simulink library "halout"  (R2021b)
settings: Solver=VariableStepAuto  StartTime=0.0  StopTime=10.0  RelTol=1e-3
undefined symbols (not defined in the file): C_TASK_5MS_S, FALSE, KHAL_CAN1FDAPS3E2E_flg, KHAL_CAN1FDAPS3TxReq_flg, KHAL_CAN1FDVCU2E2E_flg, KHAL_CAN1FDVCU2TxReq_flg, KHAL_CAN1FDVCU3E2E_flg, KHAL_CAN1FDVCU3TxReq_flg, KHAL_CAN1TxReq_flg, KHAL_CAN2TxReq_flg, KHAL_CAN3FDVCU1TxReq_flg, KHAL_CAN3FDVCU2E2E_flg, KHAL_CAN3FDVCU2TxReq_flg, KHAL_CAN3TxReq_flg, KHAL_CAN4FDVCU1E2E_flg, KHAL_CAN4FDVCU1TxReq_flg, KHAL_CAN4TxReq_flg, KHAL_CAN5TxReq_flg, ONE_INT, TRUE, ZERO_INT
libraries: FVT_lib x383, simulink x179
(part 17 of 20)

== system halout/HAL_OUT/CAN3/FD_VCU2_0x154/Byte_15 ==
  Rr_TMTqReq : Inport
  BitwiseOR : simulink/Logic and Bit Operations/Bitwise Operator  logicop=OR  UseBitMask=off  BitMask=bin2dec('11011001')  BitMaskRealWorld=Stored Integer
  SignalPack : FVT_lib/hal/SignalPack  RightShiftCnt=0  BitMask=2^8-1  LeftShiftCnt=0
  UnitConverter : DataTypeConversion  OutDataTypeStr=uint8  RndMeth=Round
  UnitConverter1 : DataTypeConversion  OutDataTypeStr=uint16  RndMeth=Round
  convert_out : FVT_lib/hal/convert_out  gain=1  offset=-530
  Byte_15 : Outport
  wires:
  BitwiseOR/1 -> Byte_15/1
  UnitConverter/1 -> BitwiseOR/1
  SignalPack/1 -> UnitConverter/1
  UnitConverter1/1 -> SignalPack/1
  convert_out/1 -> UnitConverter1/1
  Rr_TMTqReq/1 -> convert_out/1

== system halout/HAL_OUT/CAN3/FD_VCU2_0x154/Byte_16 ==
  Fr_TMTqReq : Inport
  BitwiseOR : simulink/Logic and Bit Operations/Bitwise Operator  logicop=OR  UseBitMask=off  BitMask=bin2dec('11011001')  BitMaskRealWorld=Stored Integer
  SignalPack : FVT_lib/hal/SignalPack  RightShiftCnt=8  BitMask=2^8-1  LeftShiftCnt=0
  UnitConverter : DataTypeConversion  OutDataTypeStr=uint8  RndMeth=Round
  UnitConverter1 : DataTypeConversion  OutDataTypeStr=uint16  RndMeth=Round
  convert_out : FVT_lib/hal/convert_out  gain=1  offset=-530
  Byte_16 : Outport
  wires:
  BitwiseOR/1 -> Byte_16/1
  UnitConverter/1 -> BitwiseOR/1
  SignalPack/1 -> UnitConverter/1
  UnitConverter1/1 -> SignalPack/1
  convert_out/1 -> UnitConverter1/1
  Fr_TMTqReq/1 -> convert_out/1

== system halout/HAL_OUT/CAN3/FD_VCU2_0x154/Byte_17 ==
  Fr_TMTqReq : Inport
  BitwiseOR : simulink/Logic and Bit Operations/Bitwise Operator  logicop=OR  UseBitMask=off  BitMask=bin2dec('11011001')  BitMaskRealWorld=Stored Integer
  SignalPack : FVT_lib/hal/SignalPack  RightShiftCnt=0  BitMask=2^8-1  LeftShiftCnt=0
  UnitConverter : DataTypeConversion  OutDataTypeStr=uint8  RndMeth=Round
  UnitConverter1 : DataTypeConversion  OutDataTypeStr=uint16  RndMeth=Round
  convert_out : FVT_lib/hal/convert_out  gain=1  offset=-530
  Byte_17 : Outport
  wires:
  BitwiseOR/1 -> Byte_17/1
  UnitConverter/1 -> BitwiseOR/1
  SignalPack/1 -> UnitConverter/1
  UnitConverter1/1 -> SignalPack/1
  convert_out/1 -> UnitConverter1/1
  Fr_TMTqReq/1 -> convert_out/1

== system halout/HAL_OUT/CAN3/FD_VCU2_0x154/Byte_18 ==
  Fr_IdcMax : Inport
  BitwiseOR : simulink/Logic and Bit Operations/Bitwise Operator  logicop=OR  UseBitMask=off  BitMask=bin2dec('11011001')  BitMaskRealWorld=Stored Integer
  SignalPack : FVT_lib/hal/SignalPack  RightShiftCnt=4  BitMask=2^8-1  LeftShiftCnt=0
  UnitConverter : DataTypeConversion  OutDataTypeStr=uint8  RndMeth=Round
  UnitConverter1 : DataTypeConversion  OutDataTypeStr=uint16  RndMeth=Round
  Byte_18 : Outport
  wires:
  BitwiseOR/1 -> Byte_18/1
  UnitConverter/1 -> BitwiseOR/1
  SignalPack/1 -> UnitConverter/1
  UnitConverter1/1 -> SignalPack/1
  Fr_IdcMax/1 -> UnitConverter1/1

== system halout/HAL_OUT/CAN3/FD_VCU2_0x154/Byte_19 ==
  Fr_IdcMax : Inport
  Fr_IdcMin : Inport  Port=2
  BitwiseOR : simulink/Logic and Bit Operations/Bitwise Operator  logicop=OR  UseBitMask=off  NumInputPorts=2  BitMask=bin2dec('11011001')  BitMaskRealWorld=Stored Integer
  SignalPack : FVT_lib/hal/SignalPack  RightShiftCnt=0  BitMask=2^4-1  LeftShiftCnt=4
  SignalPack1 : FVT_lib/hal/SignalPack  RightShiftCnt=8  BitMask=2^4-1  LeftShiftCnt=0
  UnitConverter : DataTypeConversion  OutDataTypeStr=uint8  RndMeth=Round
  UnitConverter1 : DataTypeConversion  OutDataTypeStr=uint16  RndMeth=Round
  UnitConverter2 : DataTypeConversion  OutDataTypeStr=uint8  RndMeth=Round
  UnitConverter3 : DataTypeConversion  OutDataTypeStr=uint16  RndMeth=Round
  convert_out : FVT_lib/hal/convert_out  gain=1  offset=-1022
  Byte_19 : Outport
  wires:
  BitwiseOR/1 -> Byte_19/1
  UnitConverter/1 -> BitwiseOR/1
  SignalPack/1 -> UnitConverter/1
  UnitConverter1/1 -> SignalPack/1
  Fr_IdcMax/1 -> UnitConverter1/1
  UnitConverter2/1 -> BitwiseOR/2
  SignalPack1/1 -> UnitConverter2/1
  UnitConverter3/1 -> SignalPack1/1
  convert_out/1 -> UnitConverter3/1
  Fr_IdcMin/1 -> convert_out/1

== system halout/HAL_OUT/CAN3/FD_VCU2_0x154/Byte_2 ==
  Rr_IdcMax : Inport
  BitwiseOR : simulink/Logic and Bit Operations/Bitwise Operator  logicop=OR  UseBitMask=off  BitMask=bin2dec('11011001')  BitMaskRealWorld=Stored Integer
  SignalPack : FVT_lib/hal/SignalPack  RightShiftCnt=4  BitMask=2^8-1  LeftShiftCnt=0
  UnitConverter : DataTypeConversion  OutDataTypeStr=uint8  RndMeth=Round
  UnitConverter1 : DataTypeConversion  OutDataTypeStr=uint16  RndMeth=Round
  Byte_2 : Outport
  wires:
  BitwiseOR/1 -> Byte_2/1
  UnitConverter/1 -> BitwiseOR/1
  SignalPack/1 -> UnitConverter/1
  UnitConverter1/1 -> SignalPack/1
  Rr_IdcMax/1 -> UnitConverter1/1

== system halout/HAL_OUT/CAN3/FD_VCU2_0x154/Byte_20 ==
  Fr_IdcMin : Inport
  BitwiseOR : simulink/Logic and Bit Operations/Bitwise Operator  logicop=OR  UseBitMask=off  BitMask=bin2dec('11011001')  BitMaskRealWorld=Stored Integer
  SignalPack : FVT_lib/hal/SignalPack  RightShiftCnt=0  BitMask=2^8-1  LeftShiftCnt=0
  UnitConverter : DataTypeConversion  OutDataTypeStr=uint8  RndMeth=Round
  UnitConverter1 : DataTypeConversion  OutDataTypeStr=uint16  RndMeth=Round
  convert_out : FVT_lib/hal/convert_out  gain=1  offset=-1022
  Byte_20 : Outport
  wires:
  BitwiseOR/1 -> Byte_20/1
  UnitConverter/1 -> BitwiseOR/1
  SignalPack/1 -> UnitConverter/1
  UnitConverter1/1 -> SignalPack/1
  convert_out/1 -> UnitConverter1/1
  Fr_IdcMin/1 -> convert_out/1

== system halout/HAL_OUT/CAN3/FD_VCU2_0x154/Byte_21 ==
  Fr_TorqMax : Inport
  BitwiseOR : simulink/Logic and Bit Operations/Bitwise Operator  logicop=OR  UseBitMask=off  BitMask=bin2dec('11011001')  BitMaskRealWorld=Stored Integer
  SignalPack : FVT_lib/hal/SignalPack  RightShiftCnt=4  BitMask=2^8-1  LeftShiftCnt=0
  UnitConverter : DataTypeConversion  OutDataTypeStr=uint8  RndMeth=Round
  UnitConverter1 : DataTypeConversion  OutDataTypeStr=uint16  RndMeth=Round
  Byte_21 : Outport
  wires:
  BitwiseOR/1 -> Byte_21/1
  UnitConverter/1 -> BitwiseOR/1
  SignalPack/1 -> UnitConverter/1
  UnitConverter1/1 -> SignalPack/1
  Fr_TorqMax/1 -> UnitConverter1/1

== system halout/HAL_OUT/CAN3/FD_VCU2_0x154/Byte_22 ==
  Fr_TorqMax : Inport
  Fr_TorqMin : Inport  Port=2
  BitwiseOR : simulink/Logic and Bit Operations/Bitwise Operator  logicop=OR  UseBitMask=off  NumInputPorts=2  BitMask=bin2dec('11011001')  BitMaskRealWorld=Stored Integer
  SignalPack : FVT_lib/hal/SignalPack  RightShiftCnt=0  BitMask=2^4-1  LeftShiftCnt=4
  SignalPack1 : FVT_lib/hal/SignalPack  RightShiftCnt=8  BitMask=2^4-1  LeftShiftCnt=0
  UnitConverter : DataTypeConversion  OutDataTypeStr=uint8  RndMeth=Round
  UnitConverter1 : DataTypeConversion  OutDataTypeStr=uint16  RndMeth=Round
  UnitConverter2 : DataTypeConversion  OutDataTypeStr=uint8  RndMeth=Round
  UnitConverter3 : DataTypeConversion  OutDataTypeStr=uint16  RndMeth=Round
  convert_out : FVT_lib/hal/convert_out  gain=1  offset=-1022
  Byte_22 : Outport
  wires:
  BitwiseOR/1 -> Byte_22/1
  UnitConverter/1 -> BitwiseOR/1
  SignalPack/1 -> UnitConverter/1
  UnitConverter1/1 -> SignalPack/1
  Fr_TorqMax/1 -> UnitConverter1/1
  UnitConverter2/1 -> BitwiseOR/2
  SignalPack1/1 -> UnitConverter2/1
  UnitConverter3/1 -> SignalPack1/1
  convert_out/1 -> UnitConverter3/1
  Fr_TorqMin/1 -> convert_out/1

== system halout/HAL_OUT/CAN3/FD_VCU2_0x154/Byte_23 ==
  Fr_TorqMin : Inport
  BitwiseOR : simulink/Logic and Bit Operations/Bitwise Operator  logicop=OR  UseBitMask=off  BitMask=bin2dec('11011001')  BitMaskRealWorld=Stored Integer
  SignalPack : FVT_lib/hal/SignalPack  RightShiftCnt=0  BitMask=2^8-1  LeftShiftCnt=0
  UnitConverter : DataTypeConversion  OutDataTypeStr=uint8  RndMeth=Round
  UnitConverter1 : DataTypeConversion  OutDataTypeStr=uint16  RndMeth=Round
  convert_out : FVT_lib/hal/convert_out  gain=1  offset=-1022
  Byte_23 : Outport
  wires:
  BitwiseOR/1 -> Byte_23/1
  UnitConverter/1 -> BitwiseOR/1
  SignalPack/1 -> UnitConverter/1
  UnitConverter1/1 -> SignalPack/1
  convert_out/1 -> UnitConverter1/1
  Fr_TorqMin/1 -> convert_out/1

== system halout/HAL_OUT/CAN3/FD_VCU2_0x154/Byte_3 ==
  Rr_IdcMax : Inport
  Rr_IdcMin : Inport  Port=2
  BitwiseOR : simulink/Logic and Bit Operations/Bitwise Operator  logicop=OR  UseBitMask=off  NumInputPorts=2  BitMask=bin2dec('11011001')  BitMaskRealWorld=Stored Integer
  SignalPack : FVT_lib/hal/SignalPack  RightShiftCnt=0  BitMask=2^4-1  LeftShiftCnt=4
  SignalPack1 : FVT_lib/hal/SignalPack  RightShiftCnt=8  BitMask=2^4-1  LeftShiftCnt=0
  UnitConverter : DataTypeConversion  OutDataTypeStr=uint8  RndMeth=Round
  UnitConverter1 : DataTypeConversion  OutDataTypeStr=uint16  RndMeth=Round
  UnitConverter2 : DataTypeConversion  OutDataTypeStr=uint8  RndMeth=Round
  UnitConverter3 : DataTypeConversion  OutDataTypeStr=uint16  RndMeth=Round
  convert_out : FVT_lib/hal/convert_out  gain=1  offset=-1022
  Byte_3 : Outport
  wires:
  BitwiseOR/1 -> Byte_3/1
  UnitConverter/1 -> BitwiseOR/1
  SignalPack/1 -> UnitConverter/1
  UnitConverter1/1 -> SignalPack/1
  Rr_IdcMax/1 -> UnitConverter1/1
  UnitConverter2/1 -> BitwiseOR/2
  SignalPack1/1 -> UnitConverter2/1
  UnitConverter3/1 -> SignalPack1/1
  convert_out/1 -> UnitConverter3/1
  Rr_IdcMin/1 -> convert_out/1

== system halout/HAL_OUT/CAN3/FD_VCU2_0x154/Byte_4 ==
  Rr_IdcMin : Inport
  BitwiseOR : simulink/Logic and Bit Operations/Bitwise Operator  logicop=OR  UseBitMask=off  BitMask=bin2dec('11011001')  BitMaskRealWorld=Stored Integer
  SignalPack : FVT_lib/hal/SignalPack  RightShiftCnt=0  BitMask=2^8-1  LeftShiftCnt=0
  UnitConverter : DataTypeConversion  OutDataTypeStr=uint8  RndMeth=Round
  UnitConverter1 : DataTypeConversion  OutDataTypeStr=uint16  RndMeth=Round
  convert_out : FVT_lib/hal/convert_out  gain=1  offset=-1022
  Byte_4 : Outport
  wires:
  BitwiseOR/1 -> Byte_4/1
  UnitConverter/1 -> BitwiseOR/1
  SignalPack/1 -> UnitConverter/1
  UnitConverter1/1 -> SignalPack/1
  convert_out/1 -> UnitConverter1/1
  Rr_IdcMin/1 -> convert_out/1

== system halout/HAL_OUT/CAN3/FD_VCU2_0x154/Byte_5 ==
  Rr_TorqMax : Inport
  BitwiseOR : simulink/Logic and Bit Operations/Bitwise Operator  logicop=OR  UseBitMask=off  BitMask=bin2dec('11011001')  BitMaskRealWorld=Stored Integer
  SignalPack : FVT_lib/hal/SignalPack  RightShiftCnt=4  BitMask=2^8-1  LeftShiftCnt=0
  UnitConverter : DataTypeConversion  OutDataTypeStr=uint8  RndMeth=Round
  UnitConverter1 : DataTypeConversion  OutDataTypeStr=uint16  RndMeth=Round
  Byte_5 : Outport
  wires:
  BitwiseOR/1 -> Byte_5/1
  UnitConverter/1 -> BitwiseOR/1
  SignalPack/1 -> UnitConverter/1
  UnitConverter1/1 -> SignalPack/1
  Rr_TorqMax/1 -> UnitConverter1/1

== system halout/HAL_OUT/CAN3/FD_VCU2_0x154/Byte_6 ==
  Rr_TorqMax : Inport
  Rr_TorqMin : Inport  Port=2
  BitwiseOR : simulink/Logic and Bit Operations/Bitwise Operator  logicop=OR  UseBitMask=off  NumInputPorts=2  BitMask=bin2dec('11011001')  BitMaskRealWorld=Stored Integer
  SignalPack : FVT_lib/hal/SignalPack  RightShiftCnt=0  BitMask=2^4-1  LeftShiftCnt=4
  SignalPack1 : FVT_lib/hal/SignalPack  RightShiftCnt=8  BitMask=2^4-1  LeftShiftCnt=0
  UnitConverter : DataTypeConversion  OutDataTypeStr=uint8  RndMeth=Round
  UnitConverter1 : DataTypeConversion  OutDataTypeStr=uint16  RndMeth=Round
  UnitConverter2 : DataTypeConversion  OutDataTypeStr=uint8  RndMeth=Round
  UnitConverter3 : DataTypeConversion  OutDataTypeStr=uint16  RndMeth=Round
  convert_out : FVT_lib/hal/convert_out  gain=1  offset=-1022
  Byte_6 : Outport
  wires:
  BitwiseOR/1 -> Byte_6/1
  UnitConverter/1 -> BitwiseOR/1
  SignalPack/1 -> UnitConverter/1
  UnitConverter1/1 -> SignalPack/1
  Rr_TorqMax/1 -> UnitConverter1/1
  UnitConverter2/1 -> BitwiseOR/2
  SignalPack1/1 -> UnitConverter2/1
  UnitConverter3/1 -> SignalPack1/1
  convert_out/1 -> UnitConverter3/1
  Rr_TorqMin/1 -> convert_out/1

== system halout/HAL_OUT/CAN3/FD_VCU2_0x154/Byte_7 ==
  Rr_TorqMin : Inport
  BitwiseOR : simulink/Logic and Bit Operations/Bitwise Operator  logicop=OR  UseBitMask=off  BitMask=bin2dec('11011001')  BitMaskRealWorld=Stored Integer
  SignalPack : FVT_lib/hal/SignalPack  RightShiftCnt=0  BitMask=2^8-1  LeftShiftCnt=0
  UnitConverter : DataTypeConversion  OutDataTypeStr=uint8  RndMeth=Round
  UnitConverter1 : DataTypeConversion  OutDataTypeStr=uint16  RndMeth=Round
  convert_out : FVT_lib/hal/convert_out  gain=1  offset=-1022
  Byte_7 : Outport
  wires:
  BitwiseOR/1 -> Byte_7/1
  UnitConverter/1 -> BitwiseOR/1
  SignalPack/1 -> UnitConverter/1
  UnitConverter1/1 -> SignalPack/1
  convert_out/1 -> UnitConverter1/1
  Rr_TorqMin/1 -> convert_out/1

== system halout/HAL_OUT/CAN3/FD_VCU2_0x154/Byte_8 ==
  Rr_UdcMax : Inport
  BitwiseOR : simulink/Logic and Bit Operations/Bitwise Operator  logicop=OR  UseBitMask=off  BitMask=bin2dec('11011001')  BitMaskRealWorld=Stored Integer
  SignalPack : FVT_lib/hal/SignalPack  RightShiftCnt=4  BitMask=2^8-1  LeftShiftCnt=0
  UnitConverter : DataTypeConversion  OutDataTypeStr=uint8  RndMeth=Round
  UnitConverter1 : DataTypeConversion  OutDataTypeStr=uint16  RndMeth=Round
  Byte_8 : Outport
  wires:
  BitwiseOR/1 -> Byte_8/1
  UnitConverter/1 -> BitwiseOR/1
  SignalPack/1 -> UnitConverter/1
  UnitConverter1/1 -> SignalPack/1
  Rr_UdcMax/1 -> UnitConverter1/1

== system halout/HAL_OUT/CAN3/FD_VCU2_0x154/Byte_9 ==
  Rr_UdcMax : Inport
  Rr_UdcMin : Inport  Port=2
  BitwiseOR : simulink/Logic and Bit Operations/Bitwise Operator  logicop=OR  UseBitMask=off  NumInputPorts=2  BitMask=bin2dec('11011001')  BitMaskRealWorld=Stored Integer
  SignalPack : FVT_lib/hal/SignalPack  RightShiftCnt=0  BitMask=2^4-1  LeftShiftCnt=4
  SignalPack1 : FVT_lib/hal/SignalPack  RightShiftCnt=8  BitMask=2^4-1  LeftShiftCnt=0
  UnitConverter : DataTypeConversion  OutDataTypeStr=uint8  RndMeth=Round
  UnitConverter1 : DataTypeConversion  OutDataTypeStr=uint16  RndMeth=Round
  UnitConverter2 : DataTypeConversion  OutDataTypeStr=uint8  RndMeth=Round
  UnitConverter3 : DataTypeConversion  OutDataTypeStr=uint16  RndMeth=Round
  Byte_9 : Outport
  wires:
  BitwiseOR/1 -> Byte_9/1
  UnitConverter/1 -> BitwiseOR/1
  SignalPack/1 -> UnitConverter/1
  UnitConverter1/1 -> SignalPack/1
  Rr_UdcMax/1 -> UnitConverter1/1
  UnitConverter2/1 -> BitwiseOR/2
  SignalPack1/1 -> UnitConverter2/1
  UnitConverter3/1 -> SignalPack1/1
  Rr_UdcMin/1 -> UnitConverter3/1

== system halout/HAL_OUT/CAN3/FD_VCU2_0x154/CSVCU2CAN1 ==
  CSVCU2CAN1 : Inport
  Data Type Conversion : DataTypeConversion  OutDataTypeStr=uint8  RndMeth=Round
  CAN3_CS_VCU2_CAN1 : Outport
  wires:
  Data Type Conversion/1 -> CAN3_CS_VCU2_CAN1/1
  CSVCU2CAN1/1 -> Data Type Conversion/1

== system halout/HAL_OUT/CAN3/FD_VCU2_0x154/FrIdcMax ==
  FrIdcMax : Inport
  Data Type Conversion : DataTypeConversion  OutDataTypeStr=uint16  RndMeth=Round
  CAN3_Fr_IdcMax : Outport
  wires:
  Data Type Conversion/1 -> CAN3_Fr_IdcMax/1
  FrIdcMax/1 -> Data Type Conversion/1

== system halout/HAL_OUT/CAN3/FD_VCU2_0x154/FrIdcMin ==
  FrIdcMin : Inport
  Data Type Conversion : DataTypeConversion  OutDataTypeStr=uint16  RndMeth=Round
  convert_out : FVT_lib/hal/convert_out  gain=1  offset=-1022
  CAN3_Fr_IdcMin : Outport
  wires:
  Data Type Conversion/1 -> CAN3_Fr_IdcMin/1
  convert_out/1 -> Data Type Conversion/1
  FrIdcMin/1 -> convert_out/1

== system halout/HAL_OUT/CAN3/FD_VCU2_0x154/FrTMTqReq ==
  FrTMTqReq : Inport
  Data Type Conversion : DataTypeConversion  OutDataTypeStr=uint16  RndMeth=Round
  convert_out : FVT_lib/hal/convert_out  gain=1  offset=-530
  CAN3_Fr_TMTqReq : Outport
  wires:
  Data Type Conversion/1 -> CAN3_Fr_TMTqReq/1
  convert_out/1 -> Data Type Conversion/1
  FrTMTqReq/1 -> convert_out/1

== system halout/HAL_OUT/CAN3/FD_VCU2_0x154/FrTorqMax ==
  FrTorqMax : Inport
  Data Type Conversion : DataTypeConversion  OutDataTypeStr=uint16  RndMeth=Round
  CAN3_Fr_TorqMax : Outport
  wires:
  Data Type Conversion/1 -> CAN3_Fr_TorqMax/1
  FrTorqMax/1 -> Data Type Conversion/1

== system halout/HAL_OUT/CAN3/FD_VCU2_0x154/FrTorqMin ==
  FrTorqMin : Inport
  Data Type Conversion : DataTypeConversion  OutDataTypeStr=uint16  RndMeth=Round
  convert_out : FVT_lib/hal/convert_out  gain=1  offset=-1022
  CAN3_Fr_TorqMin : Outport
  wires:
  Data Type Conversion/1 -> CAN3_Fr_TorqMin/1
  convert_out/1 -> Data Type Conversion/1
  FrTorqMin/1 -> convert_out/1

== system halout/HAL_OUT/CAN3/FD_VCU2_0x154/FrUdcMax ==
  FrUdcMax : Inport
  Data Type Conversion : DataTypeConversion  OutDataTypeStr=uint16  RndMeth=Round
  CAN3_Fr_UdcMax : Outport
  wires:
  Data Type Conversion/1 -> CAN3_Fr_UdcMax/1
  FrUdcMax/1 -> Data Type Conversion/1

== system halout/HAL_OUT/CAN3/FD_VCU2_0x154/FrUdcMin ==
  FrUdcMin : Inport
  Data Type Conversion : DataTypeConversion  OutDataTypeStr=uint16  RndMeth=Round
  CAN3_Fr_UdcMin : Outport
  wires:
  Data Type Conversion/1 -> CAN3_Fr_UdcMin/1
  FrUdcMin/1 -> Data Type Conversion/1

== system halout/HAL_OUT/CAN3/FD_VCU2_0x154/RCVCU2CAN1 ==
  RCVCU2CAN1 : Inport
  Data Type Conversion : DataTypeConversion  OutDataTypeStr=uint8  RndMeth=Round
  CAN3_RC_VCU2_CAN1 : Outport
  wires:
  Data Type Conversion/1 -> CAN3_RC_VCU2_CAN1/1
  RCVCU2CAN1/1 -> Data Type Conversion/1

== system halout/HAL_OUT/CAN3/FD_VCU2_0x154/RrIdcMax ==
  RrIdcMax : Inport
  Data Type Conversion : DataTypeConversion  OutDataTypeStr=uint16  RndMeth=Round
  CAN3_Rr_IdcMax : Outport
  wires:
  Data Type Conversion/1 -> CAN3_Rr_IdcMax/1
  RrIdcMax/1 -> Data Type Conversion/1

== system halout/HAL_OUT/CAN3/FD_VCU2_0x154/RrIdcMin ==
  RrIdcMin : Inport
  Data Type Conversion : DataTypeConversion  OutDataTypeStr=uint16  RndMeth=Round
  convert_out : FVT_lib/hal/convert_out  gain=1  offset=-1022
  CAN3_Rr_IdcMin : Outport
  wires:
  Data Type Conversion/1 -> CAN3_Rr_IdcMin/1
  convert_out/1 -> Data Type Conversion/1
  RrIdcMin/1 -> convert_out/1

== system halout/HAL_OUT/CAN3/FD_VCU2_0x154/RrTMTqReq ==
  RrTMTqReq : Inport
  Data Type Conversion : DataTypeConversion  OutDataTypeStr=uint16  RndMeth=Round
  convert_out : FVT_lib/hal/convert_out  gain=1  offset=-530
  CAN3_Rr_TMTqReq : Outport
  wires:
  Data Type Conversion/1 -> CAN3_Rr_TMTqReq/1
  convert_out/1 -> Data Type Conversion/1
  RrTMTqReq/1 -> convert_out/1

== system halout/HAL_OUT/CAN3/FD_VCU2_0x154/RrTorqMax ==
  RrTorqMax : Inport
  Data Type Conversion : DataTypeConversion  OutDataTypeStr=uint16  RndMeth=Round
  CAN3_Rr_TorqMax : Outport
  wires:
  Data Type Conversion/1 -> CAN3_Rr_TorqMax/1
  RrTorqMax/1 -> Data Type Conversion/1

== system halout/HAL_OUT/CAN3/FD_VCU2_0x154/RrTorqMin ==
  RrTorqMin : Inport
  Data Type Conversion : DataTypeConversion  OutDataTypeStr=uint16  RndMeth=Round
  convert_out : FVT_lib/hal/convert_out  gain=1  offset=-1022
  CAN3_Rr_TorqMin : Outport
  wires:
  Data Type Conversion/1 -> CAN3_Rr_TorqMin/1
  convert_out/1 -> Data Type Conversion/1
  RrTorqMin/1 -> convert_out/1

== system halout/HAL_OUT/CAN3/FD_VCU2_0x154/RrUdcMax ==
  RrUdcMax : Inport
  Data Type Conversion : DataTypeConversion  OutDataTypeStr=uint16  RndMeth=Round
  CAN3_Rr_UdcMax : Outport
  wires:
  Data Type Conversion/1 -> CAN3_Rr_UdcMax/1
  RrUdcMax/1 -> Data Type Conversion/1

== system halout/HAL_OUT/CAN3/FD_VCU2_0x154/RrUdcMin ==
  RrUdcMin : Inport
  Data Type Conversion : DataTypeConversion  OutDataTypeStr=uint16  RndMeth=Round
  CAN3_Rr_UdcMin : Outport
  wires:
  Data Type Conversion/1 -> CAN3_Rr_UdcMin/1
  RrUdcMin/1 -> Data Type Conversion/1

== system halout/HAL_OUT/CAN4/FD_DKC1_0x253/ApproachUnlockSW ==
  ApproachUnlockSW : Inport
  Data Type Conversion : DataTypeConversion  OutDataTypeStr=uint8  RndMeth=Round
  CAN4_Approach_Unlock_SW : Outport
  wires:
  Data Type Conversion/1 -> CAN4_Approach_Unlock_SW/1
  ApproachUnlockSW/1 -> Data Type Conversion/1

== system halout/HAL_OUT/CAN4/FD_DKC1_0x253/BrkPedalPos ==
  BrkPedalPos : Inport
  Data Type Conversion : DataTypeConversion  OutDataTypeStr=uint8  RndMeth=Round
  convert_out : FVT_lib/hal/convert_out  gain=0.4  offset=0
  CAN4_BrkPedalPos : Outport
  wires:
  Data Type Conversion/1 -> CAN4_BrkPedalPos/1
  convert_out/1 -> Data Type Conversion/1
  BrkPedalPos/1 -> convert_out/1

== system halout/HAL_OUT/CAN4/FD_DKC1_0x253/BrkPedalPosSta ==
  BrkPedalPosSta : Inport
  Data Type Conversion : DataTypeConversion  OutDataTypeStr=uint8  RndMeth=Round
  CAN4_BrkPedalPos_Sta : Outport
  wires:
  Data Type Conversion/1 -> CAN4_BrkPedalPos_Sta/1
  BrkPedalPosSta/1 -> Data Type Conversion/1

== system halout/HAL_OUT/CAN4/FD_DKC1_0x253/BrkSwSta ==
  BrkSwSta : Inport
  Data Type Conversion : DataTypeConversion  OutDataTypeStr=uint8  RndMeth=Round
  CAN4_BrkSw_Sta : Outport
  wires:
  Data Type Conversion/1 -> CAN4_BrkSw_Sta/1
  BrkSwSta/1 -> Data Type Conversion/1

== system halout/HAL_OUT/CAN4/FD_DKC1_0x253/BrkSwV ==
  BrkSwV : Inport
  Data Type Conversion : DataTypeConversion  OutDataTypeStr=uint8  RndMeth=Round
  CAN4_BrkSw_V : Outport
  wires:
  Data Type Conversion/1 -> CAN4_BrkSw_V/1
  BrkSwV/1 -> Data Type Conversion/1

== system halout/HAL_OUT/CAN4/FD_DKC1_0x253/DSEATantiset ==
  DSEATantiset : Inport
  Data Type Conversion : DataTypeConversion  OutDataTypeStr=uint8  RndMeth=Round
  CAN4_DSEAT_anti_set : Outport
  wires:
  Data Type Conversion/1 -> CAN4_DSEAT_anti_set/1
  DSEATantiset/1 -> Data Type Conversion/1

== system halout/HAL_OUT/CAN4/FD_DKC1_0x253/DSEATentryfunset ==
  DSEATentryfunset : Inport
  Data Type Conversion : DataTypeConversion  OutDataTypeStr=uint8  RndMeth=Round
  CAN4_DSEAT_entryfun_set : Outport
  wires:
  Data Type Conversion/1 -> CAN4_DSEAT_entryfun_set/1
  DSEATentryfunset/1 -> Data Type Conversion/1

== system halout/HAL_OUT/CAN4/FD_DKC1_0x253/DSEATventreq ==
  DSEATventreq : Inport
  Data Type Conversion : DataTypeConversion  OutDataTypeStr=uint8  RndMeth=Round
  CAN4_DSEAT_vent_req : Outport
  wires:
  Data Type Conversion/1 -> CAN4_DSEAT_vent_req/1
  DSEATventreq/1 -> Data Type Conversion/1

== system halout/HAL_OUT/CAN4/FD_DKC1_0x253/FDCBCMATCtrlCmd ==
  FDCBCMATCtrlCmd : Inport
  Data Type Conversion : DataTypeConversion  OutDataTypeStr=uint8  RndMeth=Round
  CAN4_FDC_BCM_ATCtrl_Cmd : Outport
  wires:
  Data Type Conversion/1 -> CAN4_FDC_BCM_ATCtrl_Cmd/1
  FDCBCMATCtrlCmd/1 -> Data Type Conversion/1

== system halout/HAL_OUT/CAN4/FD_DKC1_0x253/FDCBCMLockAlarmCmd ==
  FDCBCMLockAlarmCmd : Inport
  Data Type Conversion : DataTypeConversion  OutDataTypeStr=uint8  RndMeth=Round
  CAN4_FDC_BCM_LockAlarm_Cmd : Outport
  wires:
  Data Type Conversion/1 -> CAN4_FDC_BCM_LockAlarm_Cmd/1
  FDCBCMLockAlarmCmd/1 -> Data Type Conversion/1

== system halout/HAL_OUT/CAN4/FD_DKC1_0x253/FDCBCMOutModeCmd ==
  FDCBCMOutModeCmd : Inport
  Data Type Conversion : DataTypeConversion  OutDataTypeStr=uint8  RndMeth=Round
  CAN4_FDC_BCM_OutMode_Cmd : Outport
  wires:
  Data Type Conversion/1 -> CAN4_FDC_BCM_OutMode_Cmd/1
  FDCBCMOutModeCmd/1 -> Data Type Conversion/1

== system halout/HAL_OUT/CAN4/FD_DKC1_0x253/FDCTHCMACTInitialCmd ==
  FDCTHCMACTInitialCmd : Inport
  Data Type Conversion : DataTypeConversion  OutDataTypeStr=uint8  RndMeth=Round
  CAN4_FDC_THCM_ACTInitial_Cmd : Outport
  wires:
  Data Type Conversion/1 -> CAN4_FDC_THCM_ACTInitial_Cmd/1
  FDCTHCMACTInitialCmd/1 -> Data Type Conversion/1

== system halout/HAL_OUT/CAN4/FD_DKC1_0x253/HeadLampSW ==
  HeadLampSW : Inport
  Data Type Conversion : DataTypeConversion  OutDataTypeStr=uint8  RndMeth=Round
  CAN4_HeadLampSW : Outport
  wires:
  Data Type Conversion/1 -> CAN4_HeadLampSW/1
  HeadLampSW/1 -> Data Type Conversion/1

== system halout/HAL_OUT/CAN4/FD_DKC1_0x253/HoodLatchSW ==
  HoodLatchSW : Inport
  Data Type Conversion : DataTypeConversion  OutDataTypeStr=uint8  RndMeth=Round
  CAN4_Hood_Latch_SW : Outport
  wires:
  Data Type Conversion/1 -> CAN4_Hood_Latch_SW/1
  HoodLatchSW/1 -> Data Type Conversion/1

== system halout/HAL_OUT/CAN4/FD_DKC1_0x253/IVIISAOffsetSpd ==
  IVIISAOffsetSpd : Inport
  Data Type Conversion : DataTypeConversion  OutDataTypeStr=uint8  RndMeth=Round
  CAN4_IVI_ISA_OffsetSpd : Outport
  wires:
  Data Type Conversion/1 -> CAN4_IVI_ISA_OffsetSpd/1
  IVIISAOffsetSpd/1 -> Data Type Conversion/1

== system halout/HAL_OUT/CAN4/FD_DKC1_0x253/IVILocatedSTA ==
  IVILocatedSTA : Inport
  Data Type Conversion : DataTypeConversion  OutDataTypeStr=uint8  RndMeth=Round
  CAN4_IVI_Located_STA : Outport
  wires:
  Data Type Conversion/1 -> CAN4_IVI_Located_STA/1
  IVILocatedSTA/1 -> Data Type Conversion/1

== system halout/HAL_OUT/CAN4/FD_DKC1_0x253/IVIPTGModeSW ==
  IVIPTGModeSW : Inport
  Data Type Conversion : DataTypeConversion  OutDataTypeStr=uint8  RndMeth=Round
  CAN4_IVI_PTG_Mode_SW : Outport
  wires:
  Data Type Conversion/1 -> CAN4_IVI_PTG_Mode_SW/1
  IVIPTGModeSW/1 -> Data Type Conversion/1

== system halout/HAL_OUT/CAN4/FD_DKC1_0x253/IVIPTGOpenHeight ==
  IVIPTGOpenHeight : Inport
  Data Type Conversion : DataTypeConversion  OutDataTypeStr=uint8  RndMeth=Round
  CAN4_IVI_PTG_Open_Height : Outport
  wires:
  Data Type Conversion/1 -> CAN4_IVI_PTG_Open_Height/1
  IVIPTGOpenHeight/1 -> Data Type Conversion/1

== system halout/HAL_OUT/CAN4/FD_DKC1_0x253/IVIPTGStaSW ==
  IVIPTGStaSW : Inport
  Data Type Conversion : DataTypeConversion  OutDataTypeStr=uint8  RndMeth=Round
  CAN4_IVI_PTG_Sta_SW : Outport
  wires:
  Data Type Conversion/1 -> CAN4_IVI_PTG_Sta_SW/1
  IVIPTGStaSW/1 -> Data Type Conversion/1

== system halout/HAL_OUT/CAN4/FD_DKC1_0x253/IVIPTGUSStaSW ==
  IVIPTGUSStaSW : Inport
  Data Type Conversion : DataTypeConversion  OutDataTypeStr=uint8  RndMeth=Round
  CAN4_IVI_PTG_USSta_SW : Outport
  wires:
  Data Type Conversion/1 -> CAN4_IVI_PTG_USSta_SW/1
  IVIPTGUSStaSW/1 -> Data Type Conversion/1

== system halout/HAL_OUT/CAN4/FD_DKC1_0x253/IVITimeCheck ==
  IVITimeCheck : Inport
  Data Type Conversion : DataTypeConversion  OutDataTypeStr=uint8  RndMeth=Round
  CAN4_IVI_Time_Check : Outport
  wires:
  Data Type Conversion/1 -> CAN4_IVI_Time_Check/1
  IVITimeCheck/1 -> Data Type Conversion/1

== system halout/HAL_OUT/CAN4/FD_DKC1_0x253/IVITimeDay ==
  IVITimeDay : Inport
  Data Type Conversion : DataTypeConversion  OutDataTypeStr=uint8  RndMeth=Round
  CAN4_IVI_Time_Day : Outport
  wires:
  Data Type Conversion/1 -> CAN4_IVI_Time_Day/1
  IVITimeDay/1 -> Data Type Conversion/1

== system halout/HAL_OUT/CAN4/FD_DKC1_0x253/IVITimeHour ==
  IVITimeHour : Inport
  Data Type Conversion : DataTypeConversion  OutDataTypeStr=uint8  RndMeth=Round
  CAN4_IVI_Time_Hour : Outport
  wires:
  Data Type Conversion/1 -> CAN4_IVI_Time_Hour/1
  IVITimeHour/1 -> Data Type Conversion/1

== system halout/HAL_OUT/CAN4/FD_DKC1_0x253/IVITimeMinute ==
  IVITimeMinute : Inport
  Data Type Conversion : DataTypeConversion  OutDataTypeStr=uint8  RndMeth=Round
  CAN4_IVI_Time_Minute : Outport
  wires:
  Data Type Conversion/1 -> CAN4_IVI_Time_Minute/1
  IVITimeMinute/1 -> Data Type Conversion/1

== system halout/HAL_OUT/CAN4/FD_DKC1_0x253/IVITimeMonth ==
  IVITimeMonth : Inport
  Data Type Conversion : DataTypeConversion  OutDataTypeStr=uint8  RndMeth=Round
  CAN4_IVI_Time_Month : Outport
  wires:
  Data Type Conversion/1 -> CAN4_IVI_Time_Month/1
  IVITimeMonth/1 -> Data Type Conversion/1

== system halout/HAL_OUT/CAN4/FD_DKC1_0x253/IVITimeSecond ==
  IVITimeSecond : Inport
  Data Type Conversion : DataTypeConversion  OutDataTypeStr=uint8  RndMeth=Round
  CAN4_IVI_Time_Second : Outport
  wires:
  Data Type Conversion/1 -> CAN4_IVI_Time_Second/1
  IVITimeSecond/1 -> Data Type Conversion/1

== system halout/HAL_OUT/CAN4/FD_DKC1_0x253/IVITimeYear ==
  IVITimeYear : Inport
  Data Type Conversion : DataTypeConversion  OutDataTypeStr=uint8  RndMeth=Round
  convert_out : FVT_lib/hal/convert_out  gain=1  offset=2000
  CAN4_IVI_Time_Year : Outport
  wires:
  Data Type Conversion/1 -> CAN4_IVI_Time_Year/1
  convert_out/1 -> Data Type Conversion/1
  IVITimeYear/1 -> convert_out/1

== system halout/HAL_OUT/CAN4/FD_DKC1_0x253/LDrvCtrlCmd ==
  LDrvCtrlCmd : Inport
  Data Type Conversion : DataTypeConversion  OutDataTypeStr=uint8  RndMeth=Round
  CAN4_L_Drv_CtrlCmd : Outport
  wires:
  Data Type Conversion/1 -> CAN4_L_Drv_CtrlCmd/1
  LDrvCtrlCmd/1 -> Data Type Conversion/1

== system halout/HAL_OUT/CAN4/FD_DKC1_0x253/LPasCtrlCmd ==
  LPasCtrlCmd : Inport
  Data Type Conversion : DataTypeConversion  OutDataTypeStr=uint8  RndMeth=Round
  CAN4_L_Pas_CtrlCmd : Outport
  wires:
  Data Type Conversion/1 -> CAN4_L_Pas_CtrlCmd/1
  LPasCtrlCmd/1 -> Data Type Conversion/1

== system halout/HAL_OUT/CAN4/FD_DKC1_0x253/LRLDCtrlCmd ==
  LRLDCtrlCmd : Inport
  Data Type Conversion : DataTypeConversion  OutDataTypeStr=uint8  RndMeth=Round
  CAN4_L_RLD_CtrlCmd : Outport
  wires:
  Data Type Conversion/1 -> CAN4_L_RLD_CtrlCmd/1
  LRLDCtrlCmd/1 -> Data Type Conversion/1

== system halout/HAL_OUT/CAN4/FD_DKC1_0x253/LRRDCtrlCmd ==
  LRRDCtrlCmd : Inport
  Data Type Conversion : DataTypeConversion  OutDataTypeStr=uint8  RndMeth=Round
  CAN4_L_RRD_CtrlCmd : Outport
  wires:
  Data Type Conversion/1 -> CAN4_L_RRD_CtrlCmd/1
  LRRDCtrlCmd/1 -> Data Type Conversion/1

== system halout/HAL_OUT/CAN4/FD_DKC1_0x253/MCPressure ==
  MCPressure : Inport
  Data Type Conversion : DataTypeConversion  OutDataTypeStr=uint16  RndMeth=Round
  convert_out : FVT_lib/hal/convert_out  gain=0.1  offset=-9.7
  CAN4_MCPressure : Outport
  wires:
  Data Type Conversion/1 -> CAN4_MCPressure/1
  convert_out/1 -> Data Type Conversion/1
  MCPressure/1 -> convert_out/1

== system halout/HAL_OUT/CAN4/FD_DKC1_0x253/MCPressureV ==
  MCPressureV : Inport
  Data Type Conversion : DataTypeConversion  OutDataTypeStr=uint8  RndMeth=Round
  CAN4_MCPressure_V : Outport
  wires:
  Data Type Conversion/1 -> CAN4_MCPressure_V/1
  MCPressureV/1 -> Data Type Conversion/1

== system halout/HAL_OUT/CAN4/FD_DKC1_0x253/OFFACMODE ==
  OFFACMODE : Inport
  Data Type Conversion : DataTypeConversion  OutDataTypeStr=uint8  RndMeth=Round
  CAN4_OFF_AC_MODE : Outport
  wires:
  Data Type Conversion/1 -> CAN4_OFF_AC_MODE/1
  OFFACMODE/1 -> Data Type Conversion/1

== system halout/HAL_OUT/CAN4/FD_DKC1_0x253/PSEATventreq ==
  PSEATventreq : Inport
  Data Type Conversion : DataTypeConversion  OutDataTypeStr=uint8  RndMeth=Round
  CAN4_PSEAT_vent_req : Outport
  wires:
  Data Type Conversion/1 -> CAN4_PSEAT_vent_req/1
  PSEATventreq/1 -> Data Type Conversion/1

== system halout/HAL_OUT/CAN4/FD_DKC1_0x253/PTGInnerSW2 ==
  PTGInnerSW2 : Inport
  Data Type Conversion : DataTypeConversion  OutDataTypeStr=uint8  RndMeth=Round
  CAN4_PTG_Inner_SW2 : Outport
  wires:
  Data Type Conversion/1 -> CAN4_PTG_Inner_SW2/1
  PTGInnerSW2/1 -> Data Type Conversion/1

== system halout/HAL_OUT/CAN4/FD_DKC1_0x253/SenstivityPosition ==
  SenstivityPosition : Inport
  Data Type Conversion : DataTypeConversion  OutDataTypeStr=uint8  RndMeth=Round
  CAN4_SenstivityPosition : Outport
  wires:
  Data Type Conversion/1 -> CAN4_SenstivityPosition/1
  SenstivityPosition/1 -> Data Type Conversion/1

== system halout/HAL_OUT/CAN4/FD_DKC1_0x253/TurnSwTimeSet ==
  TurnSwTimeSet : Inport
  Data Type Conversion : DataTypeConversion  OutDataTypeStr=uint8  RndMeth=Round
  CAN4_TurnSwTimeSet : Outport
  wires:
  Data Type Conversion/1 -> CAN4_TurnSwTimeSet/1
  TurnSwTimeSet/1 -> Data Type Conversion/1

== system halout/HAL_OUT/CAN4/FD_DKC1_0x253/WalkawayLockSW ==
  WalkawayLockSW : Inport
  Data Type Conversion : DataTypeConversion  OutDataTypeStr=uint8  RndMeth=Round
  CAN4_Walkaway_Lock_SW : Outport
  wires:
  Data Type Conversion/1 -> CAN4_Walkaway_Lock_SW/1
  WalkawayLockSW/1 -> Data Type Conversion/1

== system halout/HAL_OUT/CAN4/FD_THCM1_0x182/BatteryMode ==
  BatteryMode : Inport
  Data Type Conversion : DataTypeConversion  OutDataTypeStr=uint8  RndMeth=Round
  CAN4_BatteryMode : Outport
  wires:
  Data Type Conversion/1 -> CAN4_BatteryMode/1
  BatteryMode/1 -> Data Type Conversion/1

== system halout/HAL_OUT/CAN4/FD_THCM1_0x182/CCUACLampSts ==
  CCUACLampSts : Inport
  Data Type Conversion : DataTypeConversion  OutDataTypeStr=uint8  RndMeth=Round
  CAN4_CCU_ACLampSts : Outport
  wires:
  Data Type Conversion/1 -> CAN4_CCU_ACLampSts/1
  CCUACLampSts/1 -> Data Type Conversion/1

== system halout/HAL_OUT/CAN4/FD_THCM1_0x182/CCUACMaxLampSts ==
  CCUACMaxLampSts : Inport
  Data Type Conversion : DataTypeConversion  OutDataTypeStr=uint8  RndMeth=Round
  CAN4_CCU_ACMaxLampSts : Outport
  wires:
  Data Type Conversion/1 -> CAN4_CCU_ACMaxLampSts/1
  CCUACMaxLampSts/1 -> Data Type Conversion/1

== system halout/HAL_OUT/CAN4/FD_THCM1_0x182/CCUAutoLampSts ==
  CCUAutoLampSts : Inport
  Data Type Conversion : DataTypeConversion  OutDataTypeStr=uint8  RndMeth=Round
  CAN4_CCU_AutoLampSts : Outport
  wires:
  Data Type Conversion/1 -> CAN4_CCU_AutoLampSts/1
  CCUAutoLampSts/1 -> Data Type Conversion/1

== system halout/HAL_OUT/CAN4/FD_THCM1_0x182/CCUAutoMidLampSts ==
  CCUAutoMidLampSts : Inport
  Data Type Conversion : DataTypeConversion  OutDataTypeStr=uint8  RndMeth=Round
  CAN4_CCU_AutoMidLampSts : Outport
  wires:
  Data Type Conversion/1 -> CAN4_CCU_AutoMidLampSts/1
  CCUAutoMidLampSts/1 -> Data Type Conversion/1

== system halout/HAL_OUT/CAN4/FD_THCM1_0x182/CCUDispalyRequest ==
  CCUDispalyRequest : Inport
  Data Type Conversion : DataTypeConversion  OutDataTypeStr=uint8  RndMeth=Round
  CAN4_CCU_Dispaly_Request : Outport
  wires:
  Data Type Conversion/1 -> CAN4_CCU_Dispaly_Request/1
  CCUDispalyRequest/1 -> Data Type Conversion/1

== system halout/HAL_OUT/CAN4/FD_THCM1_0x182/CCUEcoSts ==
  CCUEcoSts : Inport
  Data Type Conversion : DataTypeConversion  OutDataTypeStr=uint8  RndMeth=Round
  CAN4_CCU_EcoSts : Outport
  wires:
  Data Type Conversion/1 -> CAN4_CCU_EcoSts/1
  CCUEcoSts/1 -> Data Type Conversion/1

== system halout/HAL_OUT/CAN4/FD_THCM1_0x182/CCUFrtOnOffLampSts ==
  CCUFrtOnOffLampSts : Inport
  Data Type Conversion : DataTypeConversion  OutDataTypeStr=uint8  RndMeth=Round
  CAN4_CCU_FrtOnOffLampSts : Outport
  wires:
  Data Type Conversion/1 -> CAN4_CCU_FrtOnOffLampSts/1
  CCUFrtOnOffLampSts/1 -> Data Type Conversion/1

== system halout/HAL_OUT/CAN4/FD_THCM1_0x182/CCUHEATMaxLampSts ==
  CCUHEATMaxLampSts : Inport
  Data Type Conversion : DataTypeConversion  OutDataTypeStr=uint8  RndMeth=Round
  CAN4_CCU_HEATMaxLampSts : Outport
  wires:
  Data Type Conversion/1 -> CAN4_CCU_HEATMaxLampSts/1
  CCUHEATMaxLampSts/1 -> Data Type Conversion/1

== system halout/HAL_OUT/CAN4/FD_THCM1_0x182/CCURrOnOffLampSts ==
  CCURrOnOffLampSts : Inport
  Data Type Conversion : DataTypeConversion  OutDataTypeStr=uint8  RndMeth=Round
  CAN4_CCU_RrOnOffLampSts : Outport
  wires:
  Data Type Conversion/1 -> CAN4_CCU_RrOnOffLampSts/1
  CCURrOnOffLampSts/1 -> Data Type Conversion/1

== system halout/HAL_OUT/CAN4/FD_THCM1_0x182/CCUSyncLampSts ==
  CCUSyncLampSts : Inport
  Data Type Conversion : DataTypeConversion  OutDataTypeStr=uint8  RndMeth=Round
  CAN4_CCU_SyncLampSts : Outport
  wires:
  Data Type Conversion/1 -> CAN4_CCU_SyncLampSts/1
  CCUSyncLampSts/1 -> Data Type Conversion/1

== system halout/HAL_OUT/CAN4/FD_THCM1_0x182/CabinMode ==
  CabinMode : Inport
  Data Type Conversion : DataTypeConversion  OutDataTypeStr=uint8  RndMeth=Round
  CAN4_CabinMode : Outport
  wires:
  Data Type Conversion/1 -> CAN4_CabinMode/1
  CabinMode/1 -> Data Type Conversion/1

== system halout/HAL_OUT/CAN4/FD_THCM1_0x182/EDriveMode ==
  EDriveMode : Inport
  Data Type Conversion : DataTypeConversion  OutDataTypeStr=uint8  RndMeth=Round
  CAN4_EDriveMode : Outport
  wires:
  Data Type Conversion/1 -> CAN4_EDriveMode/1
  EDriveMode/1 -> Data Type Conversion/1

== system halout/HAL_OUT/CAN4/FD_THCM1_0x182/FDAGSCmd ==
  FDAGSCmd : Inport
  Data Type Conversion : DataTypeConversion  OutDataTypeStr=uint8  RndMeth=Round
  CAN4_FD_AGS_Cmd : Outport
  wires:
  Data Type Conversion/1 -> CAN4_FD_AGS_Cmd/1
  FDAGSCmd/1 -> Data Type Conversion/1

== system halout/HAL_OUT/CAN4/FD_THCM1_0x182/FDRecyAutoCmd ==
  FDRecyAutoCmd : Inport
  Data Type Conversion : DataTypeConversion  OutDataTypeStr=uint8  RndMeth=Round
  CAN4_FD_RecyAuto_Cmd : Outport
  wires:
  Data Type Conversion/1 -> CAN4_FD_RecyAuto_Cmd/1
  FDRecyAutoCmd/1 -> Data Type Conversion/1

== system halout/HAL_OUT/CAN4/FD_THCM1_0x182/FrCoolantflow ==
  FrCoolantflow : Inport
  Data Type Conversion : DataTypeConversion  OutDataTypeStr=uint8  RndMeth=Round
  convert_out : FVT_lib/hal/convert_out  gain=0.25  offset=0
  CAN4_Fr_Coolantflow : Outport
  wires:
  Data Type Conversion/1 -> CAN4_Fr_Coolantflow/1
  convert_out/1 -> Data Type Conversion/1
  FrCoolantflow/1 -> convert_out/1

== system halout/HAL_OUT/CAN4/FD_THCM1_0x182/FrCoolanttemp ==
  FrCoolanttemp : Inport
  Data Type Conversion : DataTypeConversion  OutDataTypeStr=uint16  RndMeth=Round
  convert_out : FVT_lib/hal/convert_out  gain=1  offset=-40
  CAN4_Fr_Coolanttemp : Outport
  wires:
  Data Type Conversion/1 -> CAN4_Fr_Coolanttemp/1
  convert_out/1 -> Data Type Conversion/1
  FrCoolanttemp/1 -> convert_out/1

== system halout/HAL_OUT/CAN4/FD_THCM1_0x182/HPThermalRecoveryReq ==
  HPThermalRecoveryReq : Inport
  Data Type Conversion : DataTypeConversion  OutDataTypeStr=uint8  RndMeth=Round
  CAN4_HPThermalRecoveryReq : Outport
  wires:
  Data Type Conversion/1 -> CAN4_HPThermalRecoveryReq/1
  HPThermalRecoveryReq/1 -> Data Type Conversion/1

== system halout/HAL_OUT/CAN4/FD_THCM1_0x182/RrCoolantflow ==
  RrCoolantflow : Inport
  Data Type Conversion : DataTypeConversion  OutDataTypeStr=uint8  RndMeth=Round
  convert_out : FVT_lib/hal/convert_out  gain=0.25  offset=0
  CAN4_Rr_Coolantflow : Outport
  wires:
  Data Type Conversion/1 -> CAN4_Rr_Coolantflow/1
  convert_out/1 -> Data Type Conversion/1
  RrCoolantflow/1 -> convert_out/1

== system halout/HAL_OUT/CAN4/FD_THCM1_0x182/RrCoolanttemp ==
  RrCoolanttemp : Inport
  Data Type Conversion : DataTypeConversion  OutDataTypeStr=uint16  RndMeth=Round
  convert_out : FVT_lib/hal/convert_out  gain=1  offset=-40
  CAN4_Rr_Coolanttemp : Outport
  wires:
  Data Type Conversion/1 -> CAN4_Rr_Coolanttemp/1
  convert_out/1 -> Data Type Conversion/1
  RrCoolanttemp/1 -> convert_out/1

== system halout/HAL_OUT/CAN4/FD_THCM1_0x182/sigAirIntenZon1St ==
  sigAirIntenZon1St : Inport
  Data Type Conversion : DataTypeConversion  OutDataTypeStr=uint8  RndMeth=Round
  CAN4_sigAirIntenZon1St : Outport
  wires:
  Data Type Conversion/1 -> CAN4_sigAirIntenZon1St/1
  sigAirIntenZon1St/1 -> Data Type Conversion/1

== system halout/HAL_OUT/CAN4/FD_THCM1_0x182/sigAirIntenZon3St ==
  sigAirIntenZon3St : Inport
  Data Type Conversion : DataTypeConversion  OutDataTypeStr=uint8  RndMeth=Round
  CAN4_sigAirIntenZon3St : Outport
  wires:
  Data Type Conversion/1 -> CAN4_sigAirIntenZon3St/1
  sigAirIntenZon3St/1 -> Data Type Conversion/1

== system halout/HAL_OUT/CAN4/FD_THCM1_0x182/sigAmbAirT ==
  sigAmbAirT : Inport
  Data Type Conversion : DataTypeConversion  OutDataTypeStr=uint8  RndMeth=Round
  convert_out : FVT_lib/hal/convert_out  gain=0.5  offset=-40
  CAN4_sigAmbAirT : Outport
  wires:
  Data Type Conversion/1 -> CAN4_sigAmbAirT/1
  convert_out/1 -> Data Type Conversion/1
  sigAmbAirT/1 -> convert_out/1

== system halout/HAL_OUT/CAN4/FD_THCM1_0x182/sigCbnAirT ==
  sigCbnAirT : Inport
  Data Type Conversion : DataTypeConversion  OutDataTypeStr=uint8  RndMeth=Round
  convert_out : FVT_lib/hal/convert_out  gain=0.5  offset=-40
  CAN4_sigCbnAirT : Outport
  wires:
  Data Type Conversion/1 -> CAN4_sigCbnAirT/1
  convert_out/1 -> Data Type Conversion/1
  sigCbnAirT/1 -> convert_out/1

== system halout/HAL_OUT/CAN4/FD_THCM1_0x182/sigCbnPTCPwrAct ==
  sigCbnPTCPwrAct : Inport
  Data Type Conversion : DataTypeConversion  OutDataTypeStr=uint8  RndMeth=Round
  convert_out : FVT_lib/hal/convert_out  gain=50  offset=0
  CAN4_sigCbnPTCPwrAct : Outport
  wires:
  Data Type Conversion/1 -> CAN4_sigCbnPTCPwrAct/1
  convert_out/1 -> Data Type Conversion/1
  sigCbnPTCPwrAct/1 -> convert_out/1

== system halout/HAL_OUT/CAN4/FD_THCM1_0x182/sigCbnSolarLeft ==
  sigCbnSolarLeft : Inport
  Data Type Conversion : DataTypeConversion  OutDataTypeStr=uint8  RndMeth=Round
  convert_out : FVT_lib/hal/convert_out  gain=5  offset=0
  CAN4_sigCbnSolarLeft : Outport
  wires:
  Data Type Conversion/1 -> CAN4_sigCbnSolarLeft/1
  convert_out/1 -> Data Type Conversion/1
  sigCbnSolarLeft/1 -> convert_out/1

== system halout/HAL_OUT/CAN4/FD_THCM1_0x182/sigCbnSolarRight ==
  sigCbnSolarRight : Inport
  Data Type Conversion : DataTypeConversion  OutDataTypeStr=uint8  RndMeth=Round
  convert_out : FVT_lib/hal/convert_out  gain=5  offset=0
  CAN4_sigCbnSolarRight : Outport
  wires:
  Data Type Conversion/1 -> CAN4_sigCbnSolarRight/1
  convert_out/1 -> Data Type Conversion/1
  sigCbnSolarRight/1 -> convert_out/1

== system halout/HAL_OUT/CAN4/FD_THCM1_0x182/sigClmtCmprPwrAct ==
  sigClmtCmprPwrAct : Inport
  Data Type Conversion : DataTypeConversion  OutDataTypeStr=uint8  RndMeth=Round
  convert_out : FVT_lib/hal/convert_out  gain=50  offset=0
  CAN4_sigClmtCmprPwrAct : Outport
  wires:
  Data Type Conversion/1 -> CAN4_sigClmtCmprPwrAct/1
  convert_out/1 -> Data Type Conversion/1
  sigClmtCmprPwrAct/1 -> convert_out/1

== system halout/HAL_OUT/CAN4/FD_THCM1_0x182/sigClntTHvBattOut ==
  sigClntTHvBattOut : Inport
  Data Type Conversion : DataTypeConversion  OutDataTypeStr=uint8  RndMeth=Round
  convert_out : FVT_lib/hal/convert_out  gain=0.5  offset=-40
  CAN4_sigClntTHvBattOut : Outport
  wires:
  Data Type Conversion/1 -> CAN4_sigClntTHvBattOut/1
  convert_out/1 -> Data Type Conversion/1
  sigClntTHvBattOut/1 -> convert_out/1

== system halout/HAL_OUT/CAN4/FD_THCM1_0x182/sigDfrstSt ==
  sigDfrstSt : Inport
  Data Type Conversion : DataTypeConversion  OutDataTypeStr=uint8  RndMeth=Round
  CAN4_sigDfrstSt : Outport
  wires:
  Data Type Conversion/1 -> CAN4_sigDfrstSt/1
  sigDfrstSt/1 -> Data Type Conversion/1

== system halout/HAL_OUT/CAN4/FD_THCM1_0x182/sigHvacSt ==
  sigHvacSt : Inport
  Data Type Conversion : DataTypeConversion  OutDataTypeStr=uint8  RndMeth=Round
  CAN4_sigHvacSt : Outport
  wires:
  Data Type Conversion/1 -> CAN4_sigHvacSt/1
  sigHvacSt/1 -> Data Type Conversion/1

== system halout/HAL_OUT/CAN4/FD_THCM1_0x182/sigRecircSt ==
  sigRecircSt : Inport
  Data Type Conversion : DataTypeConversion  OutDataTypeStr=uint8  RndMeth=Round
  CAN4_sigRecircSt : Outport
  wires:
  Data Type Conversion/1 -> CAN4_sigRecircSt/1
  sigRecircSt/1 -> Data Type Conversion/1

== system halout/HAL_OUT/CAN4/FD_THCM1_0x182/sigSetTempZon1St ==
  sigSetTempZon1St : Inport
  Data Type Conversion : DataTypeConversion  OutDataTypeStr=uint8  RndMeth=Round
  convert_out : FVT_lib/hal/convert_out  gain=0.5  offset=17
  CAN4_sigSetTempZon1St : Outport
  wires:
  Data Type Conversion/1 -> CAN4_sigSetTempZon1St/1
  convert_out/1 -> Data Type Conversion/1
  sigSetTempZon1St/1 -> convert_out/1

== system halout/HAL_OUT/CAN4/FD_THCM1_0x182/sigSetTempZon2St ==
  sigSetTempZon2St : Inport
  Data Type Conversion : DataTypeConversion  OutDataTypeStr=uint8  RndMeth=Round
  convert_out : FVT_lib/hal/convert_out  gain=0.5  offset=17
  CAN4_sigSetTempZon2St : Outport
  wires:
  Data Type Conversion/1 -> CAN4_sigSetTempZon2St/1
  convert_out/1 -> Data Type Conversion/1
  sigSetTempZon2St/1 -> convert_out/1

== system halout/HAL_OUT/CAN4/FD_THCM1_0x182/sigSetTempZon3St ==
  sigSetTempZon3St : Inport
  Data Type Conversion : DataTypeConversion  OutDataTypeStr=uint8  RndMeth=Round
  convert_out : FVT_lib/hal/convert_out  gain=0.5  offset=17
  CAN4_sigSetTempZon3St : Outport
  wires:
  Data Type Conversion/1 -> CAN4_sigSetTempZon3St/1
  convert_out/1 -> Data Type Conversion/1
  sigSetTempZon3St/1 -> convert_out/1

== system halout/HAL_OUT/CAN4/FD_THCM1_0x182/sigWindDirZon1St ==
  sigWindDirZon1St : Inport
  Data Type Conversion : DataTypeConversion  OutDataTypeStr=uint8  RndMeth=Round
  CAN4_sigWindDirZon1St : Outport
  wires:
  Data Type Conversion/1 -> CAN4_sigWindDirZon1St/1
  sigWindDirZon1St/1 -> Data Type Conversion/1

== system halout/HAL_OUT/CAN4/FD_THCM1_0x182/sigWindDirZon3St ==
  sigWindDirZon3St : Inport
  Data Type Conversion : DataTypeConversion  OutDataTypeStr=uint8  RndMeth=Round
  CAN4_sigWindDirZon3St : Outport
  wires:
  Data Type Conversion/1 -> CAN4_sigWindDirZon3St/1
  sigWindDirZon3St/1 -> Data Type Conversion/1

== system halout/HAL_OUT/CAN4/FD_THCM2_0x186/ACSubMode ==
  ACSubMode : Inport
  Data Type Conversion : DataTypeConversion  OutDataTypeStr=uint8  RndMeth=Round
  CAN4_ACSubMode : Outport
  wires:
  Data Type Conversion/1 -> CAN4_ACSubMode/1
  ACSubMode/1 -> Data Type Conversion/1

== system halout/HAL_OUT/CAN4/FD_THCM2_0x186/APTCActFrRiPwr ==
  APTCActFrRiPwr : Inport
  Data Type Conversion : DataTypeConversion  OutDataTypeStr=uint8  RndMeth=Round
  convert_out : FVT_lib/hal/convert_out  gain=25  offset=0
  CAN4_APTC_ActFrRiPwr : Outport
  wires:
  Data Type Conversion/1 -> CAN4_APTC_ActFrRiPwr/1
  convert_out/1 -> Data Type Conversion/1
  APTCActFrRiPwr/1 -> convert_out/1

== system halout/HAL_OUT/CAN4/FD_THCM2_0x186/BatLoopActWtFlw ==
  BatLoopActWtFlw : Inport
  Data Type Conversion : DataTypeConversion  OutDataTypeStr=uint8  RndMeth=Round
  convert_out : FVT_lib/hal/convert_out  gain=0.1  offset=-5
  CAN4_BatLoopActWtFlw : Outport
  wires:
  Data Type Conversion/1 -> CAN4_BatLoopActWtFlw/1
  convert_out/1 -> Data Type Conversion/1
  BatLoopActWtFlw/1 -> convert_out/1

== system halout/HAL_OUT/CAN4/FD_THCM2_0x186/CCUCbnPreACWkSts ==
  CCUCbnPreACWkSts : Inport
  Data Type Conversion : DataTypeConversion  OutDataTypeStr=uint8  RndMeth=Round
  CAN4_CCU_CbnPreACWkSts : Outport
  wires:
  Data Type Conversion/1 -> CAN4_CCU_CbnPreACWkSts/1
  CCUCbnPreACWkSts/1 -> Data Type Conversion/1

== system halout/HAL_OUT/CAN4/FD_THCM2_0x186/CCUCbnPreEstimdTi ==
  CCUCbnPreEstimdTi : Inport
  Data Type Conversion : DataTypeConversion  OutDataTypeStr=uint8  RndMeth=Round
  CAN4_CCU_CbnPreEstimdTi : Outport
  wires:
  Data Type Conversion/1 -> CAN4_CCU_CbnPreEstimdTi/1
  CCUCbnPreEstimdTi/1 -> Data Type Conversion/1

== system halout/HAL_OUT/CAN4/FD_THCM2_0x186/CCUCbnPreSts ==
  CCUCbnPreSts : Inport
  Data Type Conversion : DataTypeConversion  OutDataTypeStr=uint8  RndMeth=Round
  CAN4_CCU_CbnPreSts : Outport
  wires:
  Data Type Conversion/1 -> CAN4_CCU_CbnPreSts/1
  CCUCbnPreSts/1 -> Data Type Conversion/1

== system halout/HAL_OUT/CAN4/FD_THCM2_0x186/CCUHiVoltageReq ==
  CCUHiVoltageReq : Inport
  Data Type Conversion : DataTypeConversion  OutDataTypeStr=uint8  RndMeth=Round
  CAN4_CCU_HiVoltageReq : Outport
  wires:
  Data Type Conversion/1 -> CAN4_CCU_HiVoltageReq/1
  CCUHiVoltageReq/1 -> Data Type Conversion/1

== system halout/HAL_OUT/CAN4/FD_THCM2_0x186/CoolgFanActDuty ==
  CoolgFanActDuty : Inport
  Data Type Conversion : DataTypeConversion  OutDataTypeStr=uint8  RndMeth=Round
  convert_out : FVT_lib/hal/convert_out  gain=0.5  offset=0
  CAN4_CoolgFanActDuty : Outport
  wires:
  Data Type Conversion/1 -> CAN4_CoolgFanActDuty/1
  convert_out/1 -> Data Type Conversion/1
  CoolgFanActDuty/1 -> convert_out/1

== system halout/HAL_OUT/CAN4/FD_THCM2_0x186/DeiceModReq ==
  DeiceModReq : Inport
  Data Type Conversion : DataTypeConversion  OutDataTypeStr=uint8  RndMeth=Round
  CAN4_DeiceModReq : Outport
  wires:
  Data Type Conversion/1 -> CAN4_DeiceModReq/1
  DeiceModReq/1 -> Data Type Conversion/1

== system halout/HAL_OUT/CAN4/FD_THCM2_0x186/FDBlowerCmd ==
  FDBlowerCmd : Inport
  Data Type Conversion : DataTypeConversion  OutDataTypeStr=uint8  RndMeth=Round
  convert_out : FVT_lib/hal/convert_out  gain=0.8  offset=0
  CAN4_FD_Blower_Cmd : Outport
  wires:
  Data Type Conversion/1 -> CAN4_FD_Blower_Cmd/1
  convert_out/1 -> Data Type Conversion/1
  FDBlowerCmd/1 -> convert_out/1

== system halout/HAL_OUT/CAN4/FD_THCM2_0x186/FDCompCmd ==
  FDCompCmd : Inport
  Data Type Conversion : DataTypeConversion  OutDataTypeStr=uint16  RndMeth=Round
  convert_out : FVT_lib/hal/convert_out  gain=0.5  offset=0
  CAN4_FD_Comp_Cmd : Outport
  wires:
  Data Type Conversion/1 -> CAN4_FD_Comp_Cmd/1
  convert_out/1 -> Data Type Conversion/1
  FDCompCmd/1 -> convert_out/1

== system halout/HAL_OUT/CAN4/FD_THCM2_0x186/FDEWP1Cmd ==
  FDEWP1Cmd : Inport
  Data Type Conversion : DataTypeConversion  OutDataTypeStr=uint8  RndMeth=Round
  CAN4_FD_EWP1_Cmd : Outport
  wires:
  Data Type Conversion/1 -> CAN4_FD_EWP1_Cmd/1
  FDEWP1Cmd/1 -> Data Type Conversion/1

== system halout/HAL_OUT/CAN4/FD_THCM2_0x186/FDEWP2Cmd ==
  FDEWP2Cmd : Inport
  Data Type Conversion : DataTypeConversion  OutDataTypeStr=uint8  RndMeth=Round
  CAN4_FD_EWP2_Cmd : Outport
  wires:
  Data Type Conversion/1 -> CAN4_FD_EWP2_Cmd/1
  FDEWP2Cmd/1 -> Data Type Conversion/1

== system halout/HAL_OUT/CAN4/FD_THCM2_0x186/FDEWP3Cmd ==
  FDEWP3Cmd : Inport
  Data Type Conversion : DataTypeConversion  OutDataTypeStr=uint8  RndMeth=Round
  CAN4_FD_EWP3_Cmd : Outport
  wires:
  Data Type Conversion/1 -> CAN4_FD_EWP3_Cmd/1
  FDEWP3Cmd/1 -> Data Type Conversion/1

== system halout/HAL_OUT/CAN4/FD_THCM2_0x186/FDEXV1Cmd ==
  FDEXV1Cmd : Inport
  Data Type Conversion : DataTypeConversion  OutDataTypeStr=uint16  RndMeth=Round
  CAN4_FD_EXV1_Cmd : Outport
  wires:
  Data Type Conversion/1 -> CAN4_FD_EXV1_Cmd/1
  FDEXV1Cmd/1 -> Data Type Conversion/1
